simulink model "Asynchronous_machine_model"  (R2020b)
settings: Solver=ode45  StartTime=0.0  StopTime=10.0  MaxStep=1e-4  RelTol=1e-3
InitFcn:
  | Ts = 5e-6;
  | f = 50;
  | Up = 127;
  | we = 2*pi*f;
  | P = 4;
  | L1r = 2e-3
  | L1s = 2e-3
  | Rs =  0.435 ;
  | Rr = 0.816 ;
  | Lm = 69.31e-3;
  | Ls = L1s+Lm;
  | Lr =L1r+Lm;
  | J =  0.089 ;
libraries: powerlib_meascontrol x4, powerlib x1
settings Model: Creator=Korai
settings DataIOCC: ReturnWorkspaceOutputs=off
settings DebuggingCC: ArithmeticOperatorsInVariantConditions=warning
settings SFSimCC: SimUseLocalCustomCode=off  CustomCodeUndefinedFunction=UseInterfaceOnly
settings RTWCC: RTWUseLocalCustomCode=off
settings CodeAppCC: StateflowObjectComments=on
settings ConfigComp: CovBoundaryAbsTol=1.0e-5
settings SimscapeCC: SimscapeNormalizeSystem=off

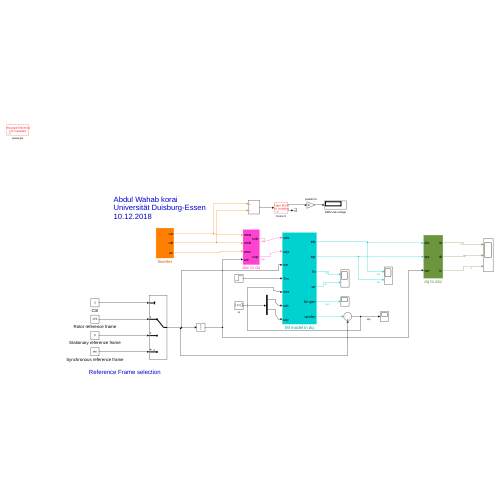
[thumbnail: Simulink's stored preview of the top-level diagram]
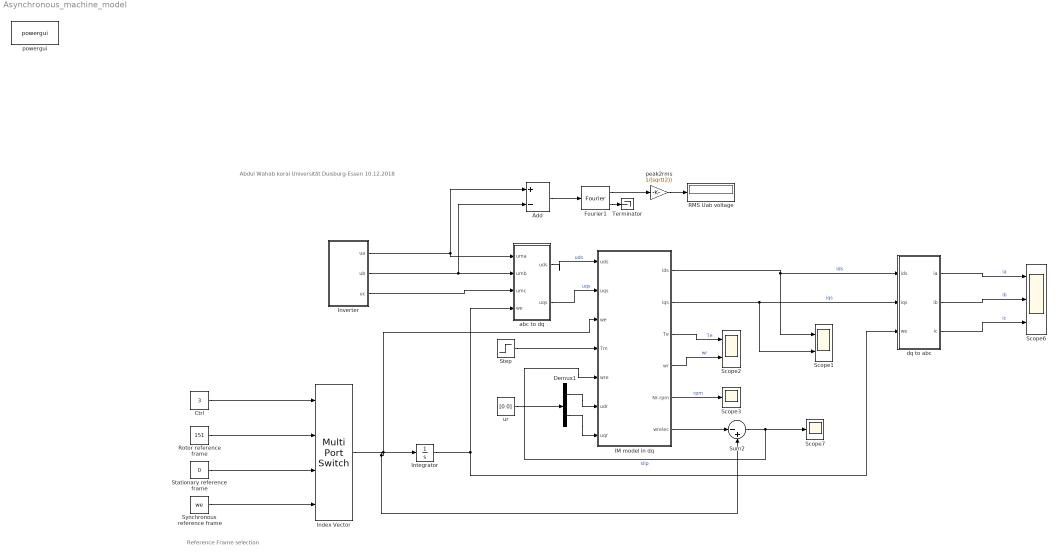
== system Asynchronous_machine_model ==
  note: Reference Frame selection
  note: Abdul Wahab korai
      | Universität Duisburg-Essen
      | 10.12.2018
  Add : Sum  Inputs=+-
  Ctrl : Constant  Value=3
  Demux1 : Demux  Outputs=2
      settings: DisplayOption=none
  Fourier1 : powerlib_meascontrol/Measurements/Fourier  Freq=50  n=1  InInit=[0, 0]  Ts=0
      settings: SourceProductName=Simscape Power Systems
  IM model in dq : Subsystem
  Index Vector : MultiPortSwitch  DataPortOrder=Specify indices
  Integrator : Integrator
  Inverter : Subsystem
  RMS Uab voltage : Display
      settings: Decimation=100
  Rotor reference frame : Constant  Value=151
  Scope1 : Scope  NumInputPorts=2
  Scope2 : Scope  NumInputPorts=2
  Scope3 : Scope
  Scope6 : Scope  NumInputPorts=3
  Scope7 : Scope
  Stationary reference frame : Constant  Value=0
  Step : Step  Time=5  After=12  SampleTime=0
  Sum2 : Sum  Inputs=|-+  SaturateOnIntegerOverflow=on
  Synchronous reference frame : Constant  Value=we
  Terminator : Terminator
  abc to dq : Subsystem
  dq to abc : Subsystem
  peak2rms : Gain  Gain=1/(sqrt(2))  SaturateOnIntegerOverflow=on  OutDataTypeStr=Inherit: Same as input  ParamDataTypeStr=Inherit: Same as input
  powergui : powerlib/powergui  Priority=1  SimulationMode=Discrete  SampleTime=Ts  frequency=60  Iterations=50  frequencyindice=50  Pbase=100e6  ErrMax=1e-4  UnitsV=kV  UnitsW=MW  buscounter=0  FunctionMessages=off  echomessages=off  EnableUseOfTLC=off  CurrentSourceSwitches=off  DisableSnubberDevices=off  DisableRonSwitches=off  DisableVfSwitches=off  DisplayEquations=off  SolverType=Tustin/Backward Euler (TBE)  Interpol=off  ExternalGateDelay=off  methode=off  Ts=100  x0status=blocks  SPID=on  SwTol=0  HookPort=off  RestoreLinks=warning  ResistiveCurrentMeasurement=off  Frange=[0:2:500]  Ylog=off  Xlog=on  ShowGrid=off  save=off  variable=ZData  structure=0  ZoomFFT=off  StartTime=0.0  cycles=1  DisplayStyle=1  fundamental=60  FreqAxis=off  MaxFrequency=1000  frequencyindicesteady=1  RmsSteady=1  display=off
  ur : Constant  Value=[0 0]
  wires:
  IM model in dq/1(ids) -> Scope1/1, dq to abc/1(ids)  "ids"
  IM model in dq/2(iqs) -> Scope1/2, dq to abc/2(iqs)  "iqs"
  abc to dq/1(uds) -> IM model in dq/1(uds)  "uds"
  abc to dq/2(uqs) -> IM model in dq/2(uqs)  "uqs"
  Step/1 -> IM model in dq/4(Tm)
  IM model in dq/4(wr) -> Scope2/2  "wr"
  IM model in dq/3(Te) -> Scope2/1  "Te"
  IM model in dq/5(Nr-rpm) -> Scope3/1  "rpm"
  dq to abc/3(ic) -> Scope6/3  "ic"
  Sum2/1 -> IM model in dq/5(wre), Scope7/1  "slip"
  Integrator/1 -> dq to abc/3(we), abc to dq/4(we)
  dq to abc/1(ia) -> Scope6/1  "ia"
  dq to abc/2(ib) -> Scope6/2  "ib"
  Fourier1/1 -> peak2rms/1
  Add/1 -> Fourier1/1
  Fourier1/2 -> Terminator/1
  peak2rms/1 -> RMS Uab voltage/1
  IM model in dq/6(wrelec) -> Sum2/1
  Demux1/1 -> IM model in dq/6(udr)
  Demux1/2 -> IM model in dq/7(uqr)
  ur/1 -> Demux1/1
  Inverter/1(ua) -> abc to dq/1(uma), Add/1
  Inverter/2(ub) -> Add/2, abc to dq/2(umb)
  Inverter/3(uc) -> abc to dq/3(umc)
  Synchronous reference frame/1 -> Index Vector/4
  Stationary reference frame/1 -> Index Vector/3
  Rotor reference frame/1 -> Index Vector/2
  Index Vector/1 -> Sum2/2, IM model in dq/3(we), Integrator/1
  Ctrl/1 -> Index Vector/1

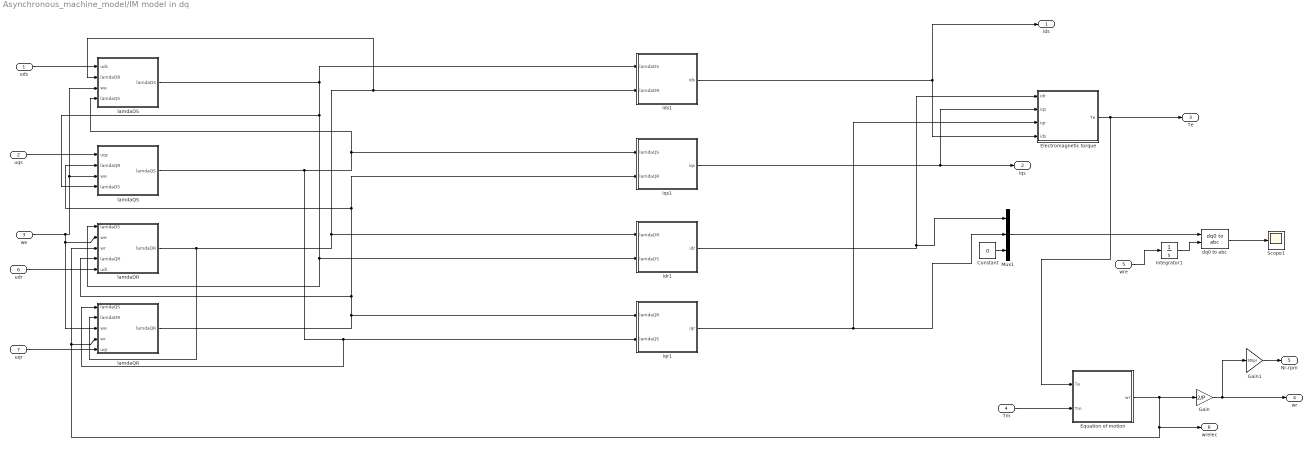
== system Asynchronous_machine_model/IM model in dq ==
  uds : Inport
  uqs : Inport  Port=2
  we : Inport  Port=3
  Tm : Inport  Port=4
  wre : Inport  Port=5
  udr : Inport  Port=6
  uqr : Inport  Port=7
  Constant : Constant  Value=0
  "Electromagnetic torque " : Subsystem
  Equation of motion : Subsystem
  Gain : Gain  Gain=2/P
  Gain1 : Gain  Gain=30/pi
  Integrator1 : Integrator
  Mux1 : Mux  Inputs=3
  Scope1 : Scope
  dq0 to abc : powerlib_meascontrol/Transformations/dq0 to abc  Alignment=90 degrees behind phase A axis
  idr1 : Subsystem
  ids1 : Subsystem
  iqr1 : Subsystem
  iqs1 : Subsystem
  lamdaDR : Subsystem
  lamdaDS : Subsystem
  lamdaQR : Subsystem
  lamdaQS : Subsystem
  ids : Outport
  iqs : Outport  Port=2
  Te : Outport  Port=3
  wr : Outport  Port=4
  Nr-rpm : Outport  Port=5
  wrelec : Outport  Port=6
  wires:
  uds/1 -> lamdaDS/1(uds)
  uqs/1 -> lamdaQS/1(uqs)
  we/1 -> lamdaQR/3(we), lamdaDR/2(we), lamdaDS/3(we), lamdaQS/3(we)
  lamdaDS/1(lamdaDS) -> lamdaQS/4(lamdaDS), lamdaDR/1(lamdaDS), idr1/2(lamdaDS), ids1/1(lamdaDS)
  lamdaDR/1(lamdaDR) -> lamdaQR/2(lamdaDR), idr1/1(lamdaDR), lamdaDS/2(lamdaDR), ids1/2(lamdaDR)
  lamdaQS/1(lamdaQS) -> lamdaQR/1(lamdaQS), iqr1/2(lamdaQS), lamdaDS/4(lamdaQS), iqs1/1(lamdaQS)
  lamdaQR/1(lamdaQR) -> iqr1/1(lamdaQR), lamdaDR/4(lamdaQR), iqs1/2(lamdaQR), lamdaQS/2(lamdaQR)
  ids1/1(ids) -> ids/1, "Electromagnetic torque "/4(ids)
  idr1/1(idr) -> "Electromagnetic torque "/1(idr), Mux1/1
  iqs1/1(iqs) -> "Electromagnetic torque "/2(iqs), iqs/1
  "Electromagnetic torque "/1(Te) -> Equation of motion/1(Te), Te/1
  Equation of motion/1(wr) -> wrelec/1, lamdaDR/3(wr), lamdaQR/4(wr), Gain/1
  Tm/1 -> Equation of motion/2(Tm)
  Gain/1 -> Gain1/1, wr/1
  Gain1/1 -> Nr-rpm/1
  iqr1/1(iqr) -> Mux1/2, "Electromagnetic torque "/3(iqr)
  Constant/1 -> Mux1/3
  Mux1/1 -> dq0 to abc/1
  dq0 to abc/1 -> Scope1/1
  wre/1 -> Integrator1/1
  Integrator1/1 -> dq0 to abc/2
  udr/1 -> lamdaDR/5(udr)
  uqr/1 -> lamdaQR/5(uqr)

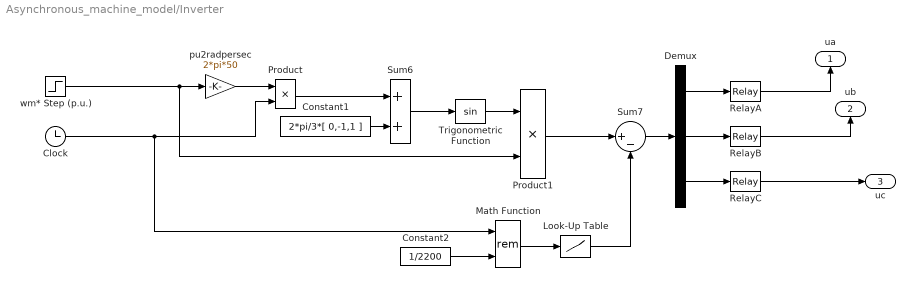
== system Asynchronous_machine_model/Inverter ==
  Clock : Clock
  Constant1 : Constant  Value=2*pi/3*[ 0,-1,1 ]
  Constant2 : Constant  Value=1/2200
  Demux : Demux  Outputs=3
      settings: DisplayOption=none
  Look-Up Table : Lookup  InputValues="[0 0.25  0.75  1] / 1980"  Table="[0  1  -1  0]"  SaturateOnIntegerOverflow=on
  Math Function : Math  Operator=rem  SignedPower=on  SaturateOnIntegerOverflow=on
  Product : Product  InputSameDT=on  SaturateOnIntegerOverflow=on  OutDataTypeStr=Inherit: Same as first input
  Product1 : Product  InputSameDT=on  SaturateOnIntegerOverflow=on  OutDataTypeStr=Inherit: Same as first input
  RelayA : Relay  OnSwitchValue=0  OffSwitchValue=0  OnOutputValue=220*sqrt(2/3)  OffOutputValue=-220*sqrt(2/3)
  RelayB : Relay  OnSwitchValue=0  OffSwitchValue=0  OnOutputValue=220*sqrt(2/3)  OffOutputValue=-220*sqrt(2/3)
  RelayC : Relay  OnSwitchValue=0  OffSwitchValue=0  OnOutputValue=220*sqrt(2/3)  OffOutputValue=-220*sqrt(2/3)
  Sum6 : Sum  InputSameDT=on  SaturateOnIntegerOverflow=on  OutDataTypeStr=Inherit: Same as first input
  Sum7 : Sum  Inputs=|+-  InputSameDT=on  SaturateOnIntegerOverflow=on  OutDataTypeStr=Inherit: Same as first input
  Trigonometric Function : Trigonometry
  pu2radpersec : Gain  Gain=2*pi*50  SaturateOnIntegerOverflow=on  OutDataTypeStr=Inherit: Same as input  ParamDataTypeStr=Inherit: Same as input
  wm* Step (p.u.) : Step  Time=0  SampleTime=0
  ua : Outport
  ub : Outport  Port=2
  uc : Outport  Port=3
  wires:
  wm* Step (p.u.)/1 -> Product1/2, pu2radpersec/1
  Constant2/1 -> Math Function/2
  RelayB/1 -> ub/1
  Demux/3 -> RelayC/1
  Constant1/1 -> Sum6/2
  Product/1 -> Sum6/1
  Product1/1 -> Sum7/1
  Demux/1 -> RelayA/1
  pu2radpersec/1 -> Product/1
  Sum6/1 -> Trigonometric Function/1
  Clock/1 -> Math Function/1, Product/2
  Trigonometric Function/1 -> Product1/1
  Demux/2 -> RelayB/1
  Sum7/1 -> Demux/1
  RelayA/1 -> ua/1
  Math Function/1 -> Look-Up Table/1
  Look-Up Table/1 -> Sum7/2
  RelayC/1 -> uc/1

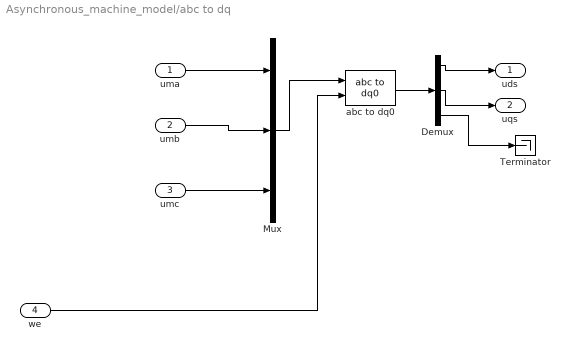
== system Asynchronous_machine_model/abc to dq ==
  uma : Inport
  umb : Inport  Port=2
  umc : Inport  Port=3
  we : Inport  Port=4
  Demux : Demux  Outputs=3
  Mux : Mux  Inputs=3
  Terminator : Terminator
  abc to dq0 : powerlib_meascontrol/Transformations/abc to dq0  Alignment=90 degrees behind phase A axis
  uds : Outport
  uqs : Outport  Port=2
  wires:
  uma/1 -> Mux/1
  Mux/1 -> abc to dq0/1
  umb/1 -> Mux/2
  umc/1 -> Mux/3
  abc to dq0/1 -> Demux/1
  Demux/1 -> uds/1
  Demux/2 -> uqs/1
  Demux/3 -> Terminator/1
  we/1 -> abc to dq0/2

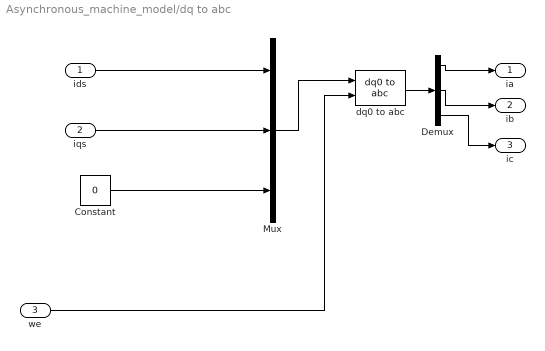
== system Asynchronous_machine_model/dq to abc ==
  ids : Inport
  iqs : Inport  Port=2
  we : Inport  Port=3
  Constant : Constant  Value=0
  Demux : Demux  Outputs=3
  Mux : Mux  Inputs=3
  dq0 to abc : powerlib_meascontrol/Transformations/dq0 to abc  Alignment=90 degrees behind phase A axis
  ia : Outport
  ib : Outport  Port=2
  ic : Outport  Port=3
  wires:
  Demux/1 -> ia/1
  Demux/2 -> ib/1
  Mux/1 -> dq0 to abc/1
  dq0 to abc/1 -> Demux/1
  Demux/3 -> ic/1
  we/1 -> dq0 to abc/2
  ids/1 -> Mux/1
  iqs/1 -> Mux/2
  Constant/1 -> Mux/3

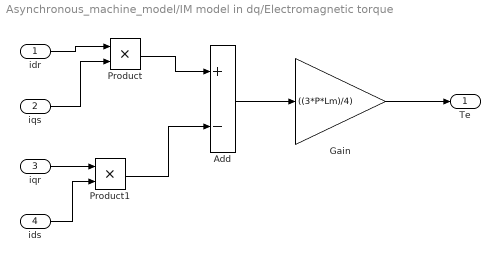
== system Asynchronous_machine_model/IM model in dq/Electromagnetic torque  ==
  idr : Inport
  iqs : Inport  Port=2
  iqr : Inport  Port=3
  ids : Inport  Port=4
  Add : Sum  Inputs=+-
  Gain : Gain  Gain=((3*P*Lm)/4)
  Product : Product
  Product1 : Product
  Te : Outport
  wires:
  idr/1 -> Product/1
  iqs/1 -> Product/2
  iqr/1 -> Product1/1
  ids/1 -> Product1/2
  Product/1 -> Add/1
  Product1/1 -> Add/2
  Gain/1 -> Te/1
  Add/1 -> Gain/1

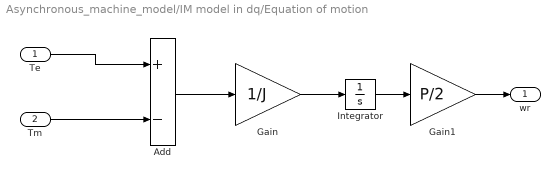
== system Asynchronous_machine_model/IM model in dq/Equation of motion ==
  Te : Inport
  Tm : Inport  Port=2
  Add : Sum  Inputs=+-
  Gain : Gain  Gain=1/J
  Gain1 : Gain  Gain=P/2
  Integrator : Integrator
  wr : Outport
  wires:
  Te/1 -> Add/1
  Tm/1 -> Add/2
  Add/1 -> Gain/1
  Gain/1 -> Integrator/1
  Integrator/1 -> Gain1/1
  Gain1/1 -> wr/1

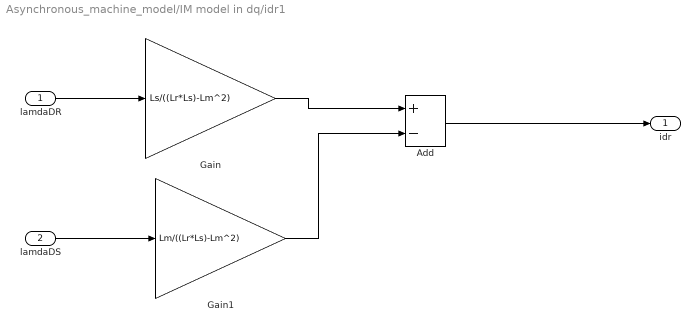
== system Asynchronous_machine_model/IM model in dq/idr1 ==
  lamdaDR : Inport
  lamdaDS : Inport  Port=2
  Add : Sum  Inputs=+-
  Gain : Gain  Gain=Ls/((Lr*Ls)-Lm^2)
  Gain1 : Gain  Gain=Lm/((Lr*Ls)-Lm^2)
  idr : Outport
  wires:
  lamdaDS/1 -> Gain1/1
  Gain/1 -> Add/1
  Gain1/1 -> Add/2
  lamdaDR/1 -> Gain/1
  Add/1 -> idr/1

== system Asynchronous_machine_model/IM model in dq/ids1 ==
  lamdaDS : Inport
  lamdaDR : Inport  Port=2
  Add : Sum  Inputs=+-
  Gain : Gain  Gain=Lr/((Lr*Ls)-Lm^2)
  Gain1 : Gain  Gain=Lm/((Lr*Ls)-Lm^2)
  ids : Outport
  wires:
  lamdaDS/1 -> Gain/1
  Add/1 -> ids/1
  Gain/1 -> Add/1
  lamdaDR/1 -> Gain1/1
  Gain1/1 -> Add/2

== system Asynchronous_machine_model/IM model in dq/iqr1 ==
  lamdaQR : Inport
  lamdaQS : Inport  Port=2
  Add : Sum  Inputs=+-
  Gain : Gain  Gain=Ls/((Lr*Ls)-Lm^2)
  Gain1 : Gain  Gain=Lm/((Lr*Ls)-Lm^2)
  iqr : Outport
  wires:
  lamdaQS/1 -> Gain1/1
  Gain/1 -> Add/1
  Gain1/1 -> Add/2
  lamdaQR/1 -> Gain/1
  Add/1 -> iqr/1

== system Asynchronous_machine_model/IM model in dq/iqs1 ==
  lamdaQS : Inport
  lamdaQR : Inport  Port=2
  Add : Sum  Inputs=+-
  Gain : Gain  Gain=Lr/((Lr*Ls)-Lm^2)
  Gain1 : Gain  Gain=Lm/((Lr*Ls)-Lm^2)
  iqs : Outport
  wires:
  lamdaQR/1 -> Gain1/1
  Gain/1 -> Add/1
  Gain1/1 -> Add/2
  lamdaQS/1 -> Gain/1
  Add/1 -> iqs/1

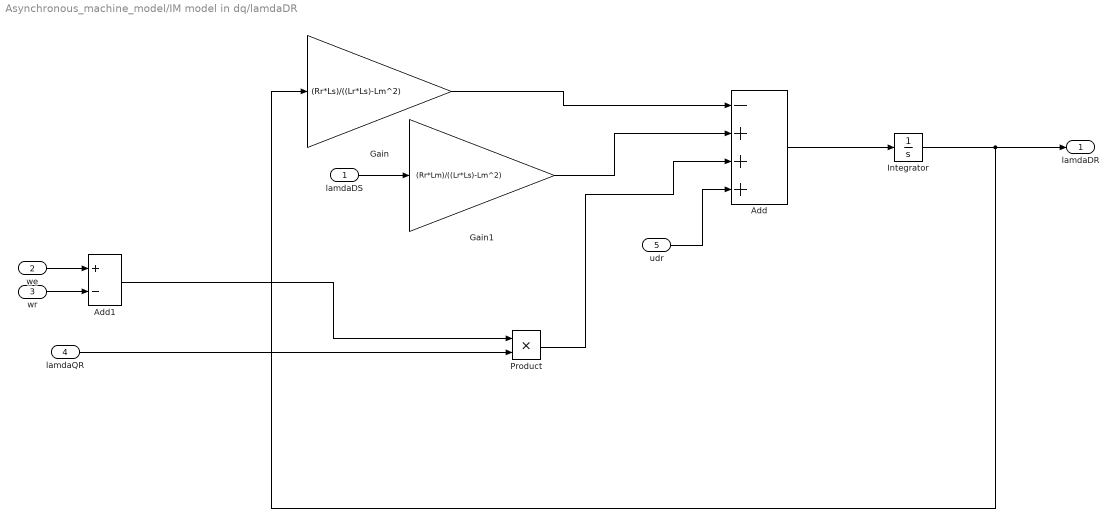
== system Asynchronous_machine_model/IM model in dq/lamdaDR ==
  lamdaDS : Inport
  we : Inport  Port=2
  wr : Inport  Port=3
  lamdaQR : Inport  Port=4
  udr : Inport  Port=5
  Add : Sum  Inputs=-+++
  Add1 : Sum  Inputs=+-
  Gain : Gain  Gain=(Rr*Ls)/((Lr*Ls)-Lm^2)
  Gain1 : Gain  Gain=(Rr*Lm)/((Lr*Ls)-Lm^2)
  Integrator : Integrator
  Product : Product
  lamdaDR : Outport
  wires:
  Add/1 -> Integrator/1
  Add1/1 -> Product/1
  lamdaQR/1 -> Product/2
  Integrator/1 -> lamdaDR/1, Gain/1
  we/1 -> Add1/1
  wr/1 -> Add1/2
  lamdaDS/1 -> Gain1/1
  Gain/1 -> Add/1
  Gain1/1 -> Add/2
  Product/1 -> Add/3
  udr/1 -> Add/4

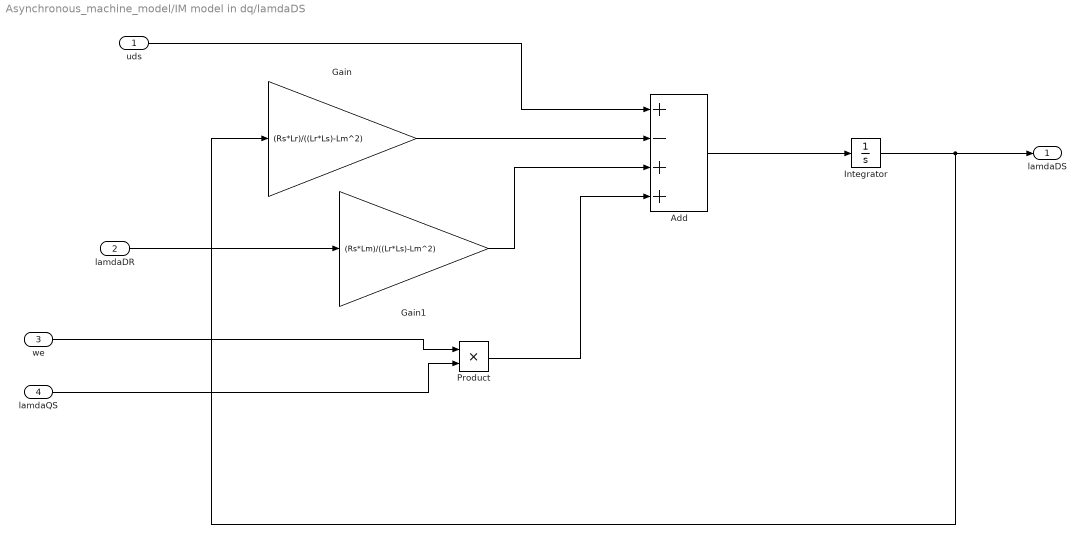
== system Asynchronous_machine_model/IM model in dq/lamdaDS ==
  uds : Inport
  lamdaDR : Inport  Port=2
  we : Inport  Port=3
  lamdaQS : Inport  Port=4
  Add : Sum  Inputs=+-++
  Gain : Gain  Gain=(Rs*Lr)/((Lr*Ls)-Lm^2)
  Gain1 : Gain  Gain=(Rs*Lm)/((Lr*Ls)-Lm^2)
  Integrator : Integrator
  Product : Product
  lamdaDS : Outport
  wires:
  uds/1 -> Add/1
  we/1 -> Product/1
  lamdaQS/1 -> Product/2
  Add/1 -> Integrator/1
  Product/1 -> Add/4
  Gain/1 -> Add/2
  Integrator/1 -> Gain/1, lamdaDS/1
  lamdaDR/1 -> Gain1/1
  Gain1/1 -> Add/3

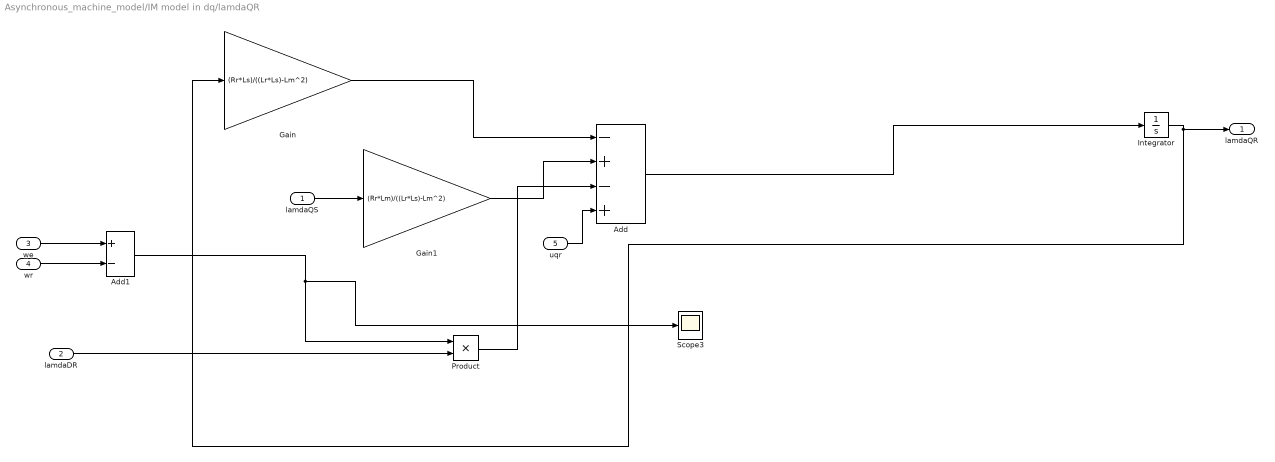
== system Asynchronous_machine_model/IM model in dq/lamdaQR ==
  lamdaQS : Inport
  lamdaDR : Inport  Port=2
  we : Inport  Port=3
  wr : Inport  Port=4
  uqr : Inport  Port=5
  Add : Sum  Inputs=-+-+
  Add1 : Sum  Inputs=+-
  Gain : Gain  Gain=(Rr*Ls)/((Lr*Ls)-Lm^2)
  Gain1 : Gain  Gain=(Rr*Lm)/((Lr*Ls)-Lm^2)
  Integrator : Integrator
  Product : Product
  Scope3 : Scope
  lamdaQR : Outport
  wires:
  lamdaQS/1 -> Gain1/1
  Add1/1 -> Scope3/1, Product/1
  Integrator/1 -> Gain/1, lamdaQR/1
  Gain1/1 -> Add/2
  lamdaDR/1 -> Product/2
  Product/1 -> Add/3
  Add/1 -> Integrator/1
  Gain/1 -> Add/1
  we/1 -> Add1/1
  wr/1 -> Add1/2
  uqr/1 -> Add/4

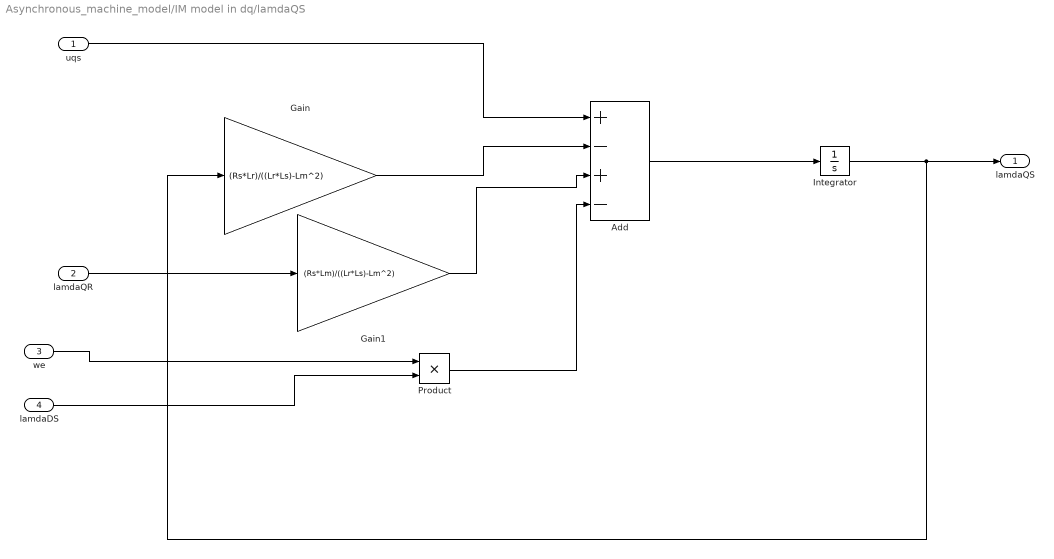
== system Asynchronous_machine_model/IM model in dq/lamdaQS ==
  uqs : Inport
  lamdaQR : Inport  Port=2
  we : Inport  Port=3
  lamdaDS : Inport  Port=4
  Add : Sum  Inputs=+-+-
  Gain : Gain  Gain=(Rs*Lr)/((Lr*Ls)-Lm^2)
  Gain1 : Gain  Gain=(Rs*Lm)/((Lr*Ls)-Lm^2)
  Integrator : Integrator
  Product : Product
  lamdaQS : Outport
  wires:
  Gain1/1 -> Add/3
  Add/1 -> Integrator/1
  uqs/1 -> Add/1
  Gain/1 -> Add/2
  we/1 -> Product/1
  lamdaQR/1 -> Gain1/1
  Product/1 -> Add/4
  lamdaDS/1 -> Product/2
  Integrator/1 -> lamdaQS/1, Gain/1
